simulink model "Beobachter_3D_Model"  (R2016b)
settings: Solver=FixedStepAuto  StartTime=0.0  StopTime=10.0  FixedStep=0.001  RelTol=1e-3
values from neighbouring files (symbols this model uses):
  A = [0, 1, 0; (m*g*l_C)/I_G, (-C_phi-C_psi)/I_G, C_psi/I_G; 0, C_psi/I_R, -C_psi/I_R]    [Beobachter_1D_diskret.m]    (also in Beobachter_3D_diskret.m = [zeros(3,3), g_LA, zeros(3,3))
  Ad = mySS.A    [Beobachter_1D_diskret.m]    (also in Beobachter_3D_diskret.m = minSYSd.A)
  B = [0; -1/I_G; 1/I_R]    [Beobachter_1D_diskret.m]    (also in Beobachter_3D_diskret.m = [zeros(3,3); -I_K_inv; I_R_inv])
  Bd = mySS.B    [Beobachter_1D_diskret.m]    (also in Beobachter_3D_diskret.m = minSYSd.B)
  C = [0, 1, 0;0,0,1]    [Beobachter_1D_diskret.m]    (also in Beobachter_3D_diskret.m = [zeros(3,3),eye(3), eye(3)])
  Cd = mySS.C    [Beobachter_1D_diskret.m]    (also in Beobachter_3D_diskret.m = minSYSd.C)
  Kd = lqrd(minSYS.A, minSYS.B, Q, R, 0.02)    [Beobachter_3D_diskret.m]
  L = (p_beo/v_beo)'    [Beobachter_3D_diskret.m]
  Ld = (place(Ad', Cd', ew_beo))'    [Beobachter_1D_diskret.m]    (also in Beobachter_3D_diskret.m)
  T_red = [eye(7), zeros(7,2)]    [Beobachter_3D_diskret.m]
  x_0 = degtorad([5;0;0])    [Beobachter_1D_diskret.m]    (also in KF_3D_linear.m = [ [-6.3118;-4.9313;-5.6638]+9.81/sqrt(3);zeros(6,1) ])
undefined symbols (not defined in the file or in its folder): minSYS, T_K
settings Model: Creator=michael  LastModifiedBy=michael

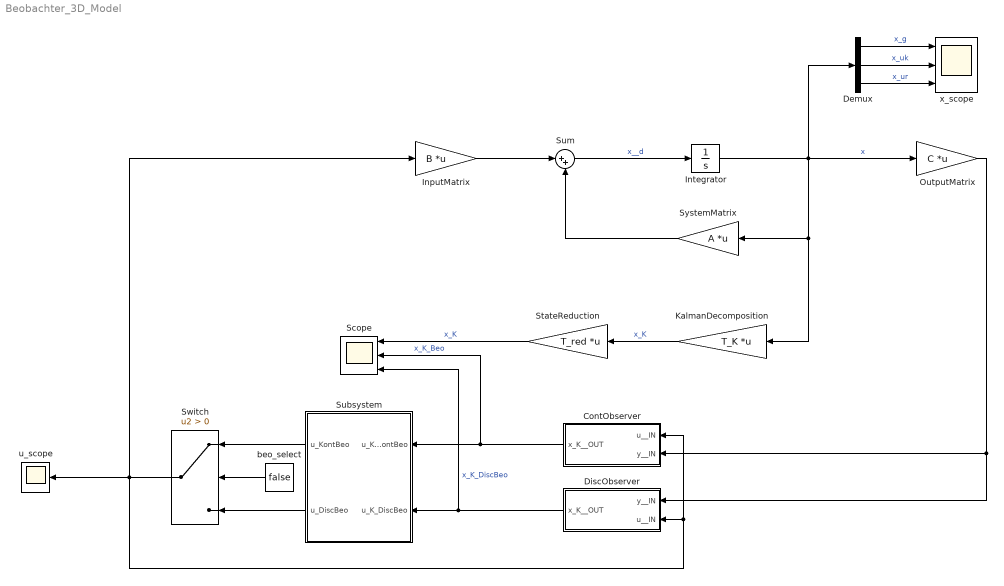
== system Beobachter_3D_Model ==
  ContObserver : Subsystem
  Demux : Demux  Outputs=3
  DiscObserver : Subsystem
  InputMatrix : Gain  Gain=B  Multiplication=Matrix(K*u) (u vector)
  Integrator : Integrator  InitialCondition=x_0
  KalmanDecomposition : Gain  Gain=T_K  Multiplication=Matrix(K*u) (u vector)
  OutputMatrix : Gain  Gain=C  Multiplication=Matrix(K*u) (u vector)
  Scope : Scope  NumInputPorts=3
  StateReduction : Gain  Gain=T_red  Multiplication=Matrix(K*u) (u vector)
  Subsystem : Subsystem
  Sum : Sum  Inputs=|++
  Switch : Switch  Criteria=u2 > Threshold
  SystemMatrix : Gain  Gain=A  Multiplication=Matrix(K*u) (u vector)
  beo_select : Constant  Value=false
  u_scope : Scope
  x_scope : Scope  NumInputPorts=3
  wires:
  Sum/1 -> Integrator/1  "x__d"
  SystemMatrix/1 -> Sum/2
  InputMatrix/1 -> Sum/1
  Integrator/1 -> Demux/1, OutputMatrix/1, KalmanDecomposition/1, SystemMatrix/1  "x"
  Demux/1 -> x_scope/1  "x_g"
  Demux/2 -> x_scope/2  "x_uk"
  Demux/3 -> x_scope/3  "x_ur"
  KalmanDecomposition/1 -> StateReduction/1  "x_K"
  OutputMatrix/1 -> DiscObserver/1(y__IN), ContObserver/2(y__IN)
  ContObserver/1(x_K__OUT) -> Scope/2, Subsystem/1(u_K_ContBeo)  "x_K_Beo"
  Switch/1 -> InputMatrix/1, u_scope/1, ContObserver/1(u__IN), DiscObserver/2(u__IN)
  beo_select/1 -> Switch/2
  Subsystem/1(u_KontBeo) -> Switch/1
  Subsystem/2(u_DiscBeo) -> Switch/3
  DiscObserver/1(x_K__OUT) -> Scope/3, Subsystem/2(u_K_DiscBeo)  "x_K_DiscBeo"
  StateReduction/1 -> Scope/1  "x_K"

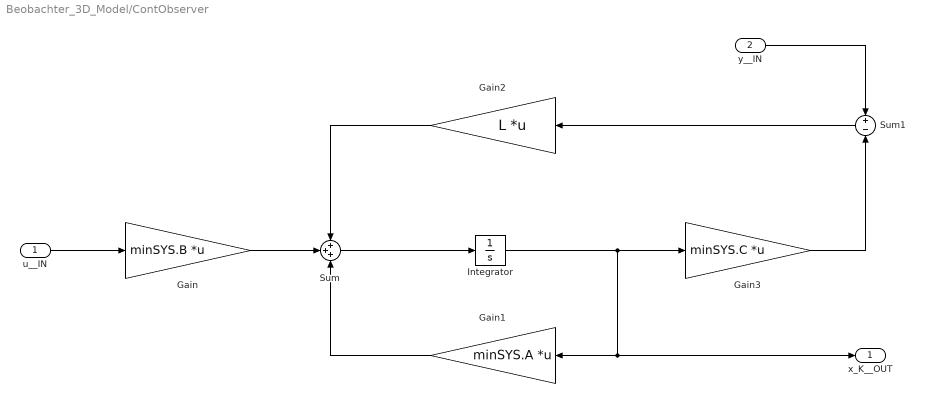
== system Beobachter_3D_Model/ContObserver ==
  u__IN : Inport
  y__IN : Inport  Port=2
  Gain : Gain  Gain=minSYS.B  Multiplication=Matrix(K*u) (u vector)
  Gain1 : Gain  Gain=minSYS.A  Multiplication=Matrix(K*u) (u vector)
  Gain2 : Gain  Gain=L  Multiplication=Matrix(K*u) (u vector)
  Gain3 : Gain  Gain=minSYS.C  Multiplication=Matrix(K*u) (u vector)
  Integrator : Integrator  InitialCondition=T_red*T_K*x_0
  Sum : Sum  Inputs=+++
  Sum1 : Sum  Inputs=+|-
  x_K__OUT : Outport
  wires:
  u__IN/1 -> Gain/1
  Gain/1 -> Sum/2
  Gain1/1 -> Sum/3
  Sum/1 -> Integrator/1
  Gain2/1 -> Sum/1
  Sum1/1 -> Gain2/1
  y__IN/1 -> Sum1/1
  Integrator/1 -> x_K__OUT/1, Gain1/1, Gain3/1
  Gain3/1 -> Sum1/2

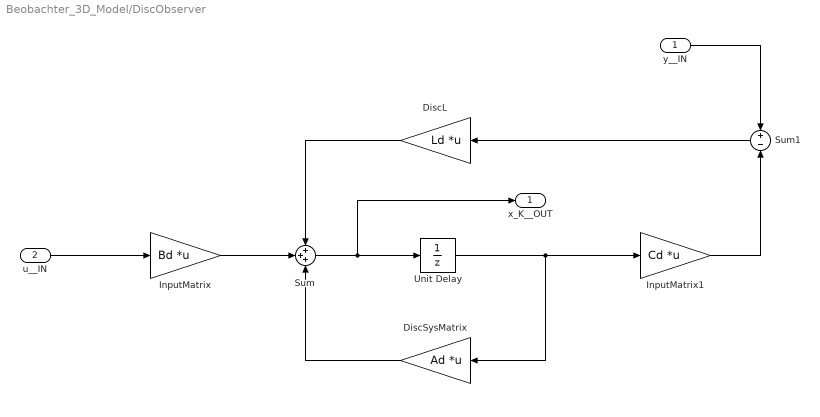
== system Beobachter_3D_Model/DiscObserver ==
  y__IN : Inport  SampleTime=0.02
  u__IN : Inport  Port=2  SampleTime=0.02
  DiscL : Gain  Gain=Ld  Multiplication=Matrix(K*u) (u vector)
  DiscSysMatrix : Gain  Gain=Ad  Multiplication=Matrix(K*u) (u vector)
  InputMatrix : Gain  Gain=Bd  Multiplication=Matrix(K*u) (u vector)
  InputMatrix1 : Gain  Gain=Cd  Multiplication=Matrix(K*u) (u vector)
  Sum : Sum  Inputs=+++
  Sum1 : Sum  Inputs=+|-
  Unit Delay : UnitDelay  InitialCondition=T_red*T_K*x_0  SampleTime=0.02
  x_K__OUT : Outport
  wires:
  u__IN/1 -> InputMatrix/1
  InputMatrix/1 -> Sum/2
  DiscSysMatrix/1 -> Sum/3
  Sum/1 -> x_K__OUT/1, Unit Delay/1
  DiscL/1 -> Sum/1
  Sum1/1 -> DiscL/1
  y__IN/1 -> Sum1/1
  InputMatrix1/1 -> Sum1/2
  Unit Delay/1 -> InputMatrix1/1, DiscSysMatrix/1

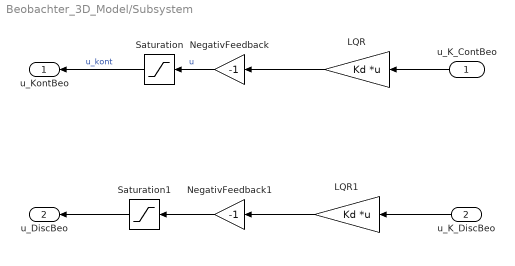
== system Beobachter_3D_Model/Subsystem ==
  u_K_ContBeo : Inport  SampleTime=0.02
  u_K_DiscBeo : Inport  Port=2  SampleTime=0.02
  LQR : Gain  Gain=Kd  Multiplication=Matrix(K*u) (u vector)
  LQR1 : Gain  Gain=Kd  Multiplication=Matrix(K*u) (u vector)
  NegativFeedback : Gain  Gain=-1
  NegativFeedback1 : Gain  Gain=-1
  Saturation : Saturate  UpperLimit=0.13  LowerLimit=-0.13
  Saturation1 : Saturate  UpperLimit=0.13  LowerLimit=-0.13
  u_KontBeo : Outport
  u_DiscBeo : Outport  Port=2
  wires:
  Saturation1/1 -> u_DiscBeo/1
  Saturation/1 -> u_KontBeo/1  "u_kont"
  NegativFeedback/1 -> Saturation/1  "u"
  u_K_ContBeo/1 -> LQR/1
  NegativFeedback1/1 -> Saturation1/1
  LQR1/1 -> NegativFeedback1/1
  LQR/1 -> NegativFeedback/1
  u_K_DiscBeo/1 -> LQR1/1
